simulink model "opv_pluto_transmitter_HDL_coder_input"  (R2023a)
settings: Solver=FixedStepDiscrete  StartTime=0.0  StopTime=.02*40e-3  RelTol=1e-3
values from neighbouring files (symbols this model uses):
  bit_rate = bits_per_symbol*symbol_rate    (= 54200)    [opv.m]
  bits_per_symbol = 2    [opv.m]
  device_clock = 61.44e6    (= 61440000)    [opv.m]
  MSK_Preamble = logical(MSK_Preamble)    [opv.m]
  PTTlength = length(PTT)    [opv.m]
  symbol_rate = 27100    [opv.m]
libraries: hdlsllib x2, dsphdlsigops2 x2, dspindex x1, commrandsrc3 x1
settings Model: Creator=matt  LastModifiedBy=matt
settings OptimizationCC: BlockReduction=off  ConditionallyExecuteInputs=off  DefaultParameterBehavior=Inlined
settings DebuggingCC: AlgebraicLoopMsg=error
settings HardwareCC: ProdBitPerPointer=32  ProdBitPerSizeT=32  ProdBitPerPtrDiffT=32  ProdLargestAtomicFloat=None  ProdIntDivRoundTo=Undefined  ProdEndianess=Unspecified  ProdWordSize=32  ProdHWDeviceType=ASIC/FPGA->ASIC/FPGA  TargetBitPerLong=64  TargetBitPerPointer=64  TargetBitPerSizeT=64  TargetBitPerPtrDiffT=64  TargetLongLongMode=on  TargetIntDivRoundTo=Zero  TargetEndianess=LittleEndian  TargetWordSize=64  TargetHWDeviceType=Custom Processor->MATLAB Host Computer  ProdEqTarget=off

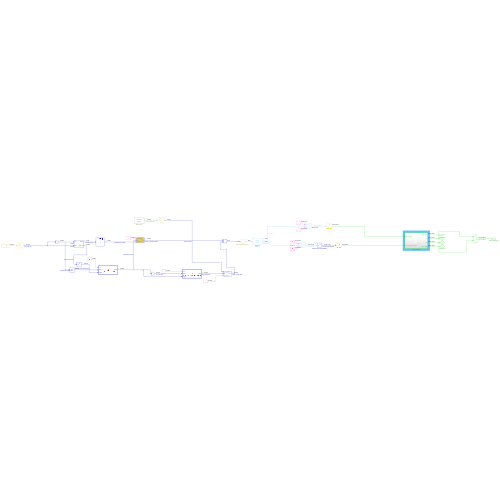
[thumbnail: Simulink's stored preview of the top-level diagram]
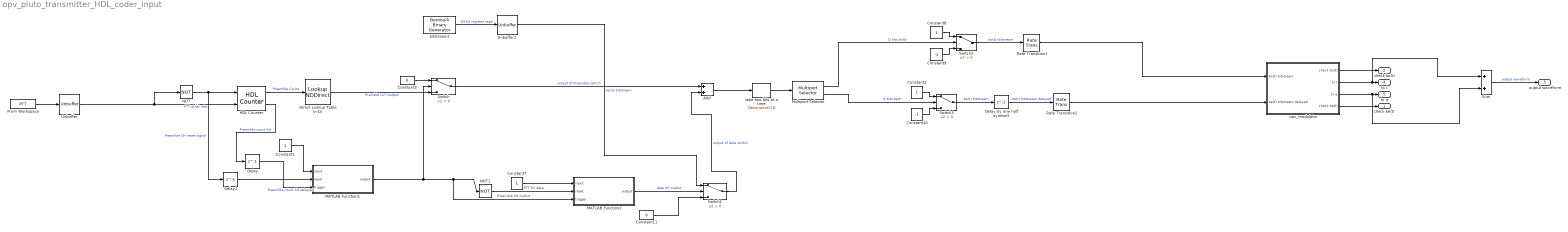
== system opv_pluto_transmitter_HDL_coder_input ==
  Add : Sum
  Constant1 : Constant  OutDataTypeStr=boolean
  Constant10 : Constant  Value=-1  OutDataTypeStr=fixdt(1,16,15)
  Constant11 : Constant  Value=0  VectorParams1D=off  OutDataTypeStr=boolean
  Constant2 : Constant  OutDataTypeStr=fixdt(1,16,15)
  Constant3 : Constant  Value=0  VectorParams1D=off  OutDataTypeStr=boolean
  Constant7 : Constant  OutDataTypeStr=boolean
  Constant8 : Constant  OutDataTypeStr=fixdt(1,16,15)
  Constant9 : Constant  Value=-1  OutDataTypeStr=fixdt(1,16,15)
  Delay : Delay  DelayLength=1
  Delay by one half symbol3 : Delay  DelayLength=1  SampleTime=1/(bits_per_symbol*symbol_rate)
  Delay1 : Delay  DelayLength=1
  Direct Lookup Table (n-D) : LookupNDDirect  NumberOfTableDimensions=1  Table=MSK_Preamble  DiagnosticForOutOfRangeInput=Error  TableDataTypeStr=boolean
  From Workspace : FromWorkspace  VariableName=PTT  SampleTime=PTTlength/(bit_rate)
  HDL Counter : hdlsllib/Sources/HDL Counter  CountType=Count limited  CountInit=0  CountStep=1  CountMax=2168  CountFromType=Initial value  CountFrom=0  CountResetPort=on  CountLoadPort=off  CountEnbPort=on  CountDirPort=off  CountHitOutputPort=on  CountDataType=Unsigned  CountWordLen=16  CountFracLen=0  CountSampTime=1
  MATLAB Function1 : MATLAB Function  TreatAsAtomicUnit=on
  MATLAB Function2 : MATLAB Function  TreatAsAtomicUnit=on
  Multiport Selector : dspindex/Multiport Selector  rowsOrCols=Rows  idxCellArray={ 1, 2 }  idxErrMode=Clip Index
      settings: LibrarySourceBlock=|
      | dsphdlsupportsigmgmt/Multiport
      | Selector
  NOT : Logic  Operator=NOT  IconShape=distinctive  AllPortsSameDT=off  OutDataTypeStr=boolean
  NOT1 : Logic  Operator=NOT  IconShape=distinctive  AllPortsSameDT=off  OutDataTypeStr=boolean
  Rate Transition1 : RateTransition  Deterministic=off  OutPortSampleTime=1/device_clock
  Rate Transition2 : RateTransition  Deterministic=off  OutPortSampleTime=1/device_clock
  Sum : Sum  OutDataTypeStr=fixdt(1,16,15)  SaturateOnIntegerOverflow=on
  Switch : Switch  Criteria=u2 > Threshold  SaturateOnIntegerOverflow=off  InputSameDT=off
  Switch1 : Switch  Criteria=u2 > Threshold  SaturateOnIntegerOverflow=off  InputSameDT=off
  Switch2 : Switch  Criteria=u2 > Threshold  OutDataTypeStr=fixdt(1,16,15)  SaturateOnIntegerOverflow=off  InputSameDT=off
  Switch3 : Switch  Criteria=u2 > Threshold  OutDataTypeStr=fixdt(1,16,15)  SaturateOnIntegerOverflow=off  InputSameDT=off
  Unbuffer : Unbuffer
  Unbuffer2 : Unbuffer
  bitstream1 : commrandsrc3/Bernoulli Binary Generator  ProbabilityOfZero=0.5  SeedSource=Auto  Seed=0  SampleTime=(1/bit_rate)  SamplesPerFrame=64  OutputDataType=boolean  SimulateUsing=Interpreted execution
  opv_modulator : Subsystem  TreatAsAtomicUnit=on
  take two bits at a time : hdlsllib/HDL Operations/Deserializer1D  Ratio=2  IdleCycles=0  InitialCondition=0  startIn=off  validIn=off  validOut=off  inputDataDimensions=-1  inputSampleTime=-1  inputSignalType=auto
  check be(t) : Outport
  "check bo(t) " : Outport  Port=2
  output waveform : Outport  Port=3
  tx I : Outport  Port=4
  tx q : Outport  Port=5
  wires:
  Switch2/1 -> Rate Transition1/1  "bo(t) bitstream"
  Switch3/1 -> Delay by one half symbol3/1  "be(t) bitstream"
  Sum/1 -> output waveform/1  "output waveform"
  Delay by one half symbol3/1 -> Rate Transition2/1  "be(t) bitstream delayed"
  Constant1/1 -> MATLAB Function1/1(input)
  Constant3/1 -> Switch/1
  HDL Counter/1 -> Direct Lookup Table (n-D)/1  "Preamble Count"
  Delay/1 -> MATLAB Function1/3(trigger)  "Preamble count hit delayed"
  MATLAB Function1/1(output) -> Switch/2, NOT1/1, MATLAB Function2/3(trigger)  "Preamble SH ouptut"
  NOT/1 -> Delay1/1, HDL Counter/1  "Preamble SH reset signal"
  Switch/1 -> Add/1  "output of Preamble switch"
  HDL Counter/2 -> Delay/1  "Preamble count hit"
  Direct Lookup Table (n-D)/1 -> Switch/3  "Premble LUT Output"
  Delay1/1 -> MATLAB Function1/2(reset)
  From Workspace/1 -> Unbuffer/1
  Unbuffer/1 -> NOT/1, HDL Counter/2  "PTT at bit rate"
  take two bits at a time/1 -> Multiport Selector/1
  Multiport Selector/1 -> Switch2/2  "Q bits bo(t)"
  Multiport Selector/2 -> Switch3/2  "Q bits be(t)"
  MATLAB Function2/1(output) -> Switch1/2  "data SH ouptut"
  NOT1/1 -> MATLAB Function2/2(reset)  "PTT for data"
  Constant7/1 -> MATLAB Function2/1(input)
  Switch1/1 -> Add/2  "output of data switch"
  Add/1 -> take two bits at a time/1
  Constant8/1 -> Switch2/1
  Constant9/1 -> Switch2/3
  Constant10/1 -> Switch3/3
  Constant2/1 -> Switch3/1
  Constant11/1 -> Switch1/3
  Unbuffer2/1 -> Switch1/1  "serial bitstream"
  bitstream1/1 -> Unbuffer2/1  "64 bit register read"
  Rate Transition1/1 -> opv_modulator/1(bo(t) bitstream)
  Rate Transition2/1 -> opv_modulator/2(be(t) bitstream delayed)
  opv_modulator/1("check bo(t) ") -> "check bo(t) "/1
  opv_modulator/2(tx I) -> Sum/1, tx I/1
  opv_modulator/3(tx q) -> Sum/2, tx q/1
  opv_modulator/4(check be(t)) -> check be(t)/1

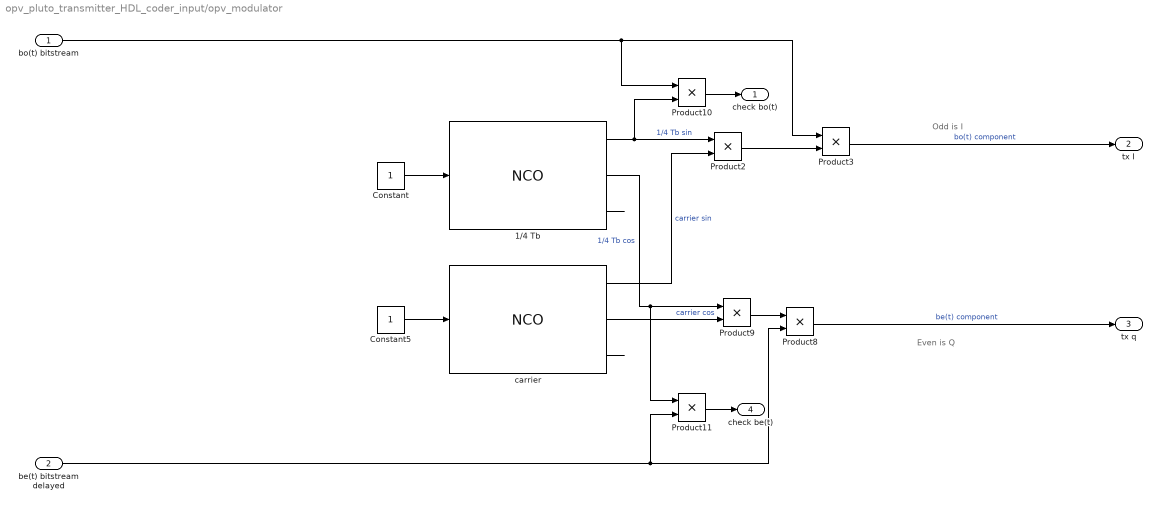
== system opv_pluto_transmitter_HDL_coder_input/opv_modulator ==
  note: Even is Q
  note: Odd is I
  bo(t) bitstream : Inport
  be(t) bitstream delayed : Inport  Port=2
  1/4 Tb : dsphdlsigops2/NCO  PhaseIncrementSource=Property  PhaseIncrement=phase_increment_bo_be  PhaseOffsetSource=Property  PhaseOffset=phase_offset  DitherSource=None  NumDitherBits=dither_bits  SamplesPerFrame=1  LUTCompress=off  ResetAction=off  Waveform=Sine and cosine  PhasePort=off  SimulateUsing=Code generation  AccumulatorWL=accumulator_width  PhaseQuantization=on  NumQuantizerAccumulatorBits=quantizer_word_length  OutputDataType=Binary point scaling  OutputWL=16  OutputFL=15
      settings: LibrarySourceBlock=dsphdlsrcs2/NCO
  Constant : Constant  OutDataTypeStr=boolean
  Constant5 : Constant  OutDataTypeStr=boolean
  Product{2..3,8..11} (6 alike) : Product  OutDataTypeStr=fixdt(1,16,15)
  carrier : dsphdlsigops2/NCO  PhaseIncrementSource=Property  PhaseIncrement=phase_increment_carrier  PhaseOffsetSource=Property  PhaseOffset=phase_offset  DitherSource=None  NumDitherBits=dither_bits  SamplesPerFrame=1  LUTCompress=off  ResetAction=off  Waveform=Sine and cosine  PhasePort=off  SimulateUsing=Code generation  AccumulatorWL=accumulator_width  PhaseQuantization=on  NumQuantizerAccumulatorBits=quantizer_word_length  OutputDataType=Binary point scaling  OutputWL=16  OutputFL=15
      settings: LibrarySourceBlock=dsphdlsrcs2/NCO
  "check bo(t) " : Outport
  tx I : Outport  Port=2
  tx q : Outport  Port=3
  check be(t) : Outport  Port=4
  wires:
  Product11/1 -> check be(t)/1
  Product10/1 -> "check bo(t) "/1
  bo(t) bitstream/1 -> Product10/1, Product3/1
  1/4 Tb/3 -> ?
  carrier/3 -> ?
  be(t) bitstream delayed/1 -> Product11/2, Product8/2
  Constant/1 -> 1/4 Tb/1
  Constant5/1 -> carrier/1
  Product8/1 -> tx q/1  "be(t) component"
  Product3/1 -> tx I/1  "bo(t) component"
  1/4 Tb/1 -> Product10/2, Product2/1  "1/4 Tb sin"
  1/4 Tb/2 -> Product11/1, Product9/1  "1/4 Tb cos"
  carrier/1 -> Product2/2  "carrier sin"
  carrier/2 -> Product9/2  "carrier cos"
  Product9/1 -> Product8/1
  Product2/1 -> Product3/2

== matlab function opv_pluto_transmitter_HDL_coder_input/MATLAB Function2 ==
  data: input input; output output; reset input; trigger input
function output   = resettable_sample_and_hold(input, reset, trigger)
%#codegen

%Resettable Sample and Hold Circuit
% This was written because S&H within Resettable Subsystems in Simulink
% is not supported by HDL Coder. We needed this functionality, so this
% custom function was written. 



initial_value = false;

    persistent sample_held;
    if isempty(sample_held)
        sample_held = false;
    end

    persistent output_held_value;
    if isempty(output_held_value)
        output_held_value = false;
    end


switch reset
    case 0 % not in reset
        switch trigger
            case 0
                output = output_held_value;
            case 1
                if sample_held == false
                    output_held_value = input;
                    output = output_held_value;
                    sample_held = true;
                else
                    output = output_held_value;
                end
            otherwise
                output = initial_value;
        end
    case 1 % reset signal received
        output = initial_value;
        sample_held = false;
        output_held_value = false;
    otherwise
        output = initial_value;
        
end

== matlab function opv_pluto_transmitter_HDL_coder_input/MATLAB Function1 ==
  data: input input; output output; reset input; trigger input
function output   = resettable_sample_and_hold(input, reset, trigger)
%#codegen

%Resettable Sample and Hold Circuit
% This was written because S&H within Resettable Subsystems in Simulink
% is not supported by HDL Coder. We needed this functionality, so this
% custom function was written. 



initial_value = false;

    persistent sample_held;
    if isempty(sample_held)
        sample_held = false;
    end

    persistent output_held_value;
    if isempty(output_held_value)
        output_held_value = false;
    end


switch reset
    case 0 % not in reset
        switch trigger
            case 0
                output = output_held_value;
            case 1
                if sample_held == false
                    output_held_value = input;
                    output = output_held_value;
                    sample_held = true;
                else
                    output = output_held_value;
                end
            otherwise
                output = initial_value;
        end
    case 1 % reset signal received
        output = initial_value;
        sample_held = false;
        output_held_value = false;
    otherwise
        output = initial_value;
        
end
